simulink model "modelref_s0"  (R2022a)
settings: Solver=FixedStepDiscrete  StartTime=0.0  StopTime=10.0  RelTol=1e-3  EnableMultiTasking=on
model workspace (MAT data in the model file):
  modelws_data = 2
settings Model: DataDictionary=modelref.sldd  Creator=KenYoshioka  LastModifiedBy=KenYoshioka
settings SolverCC: AutoInsertRateTranBlk=on
settings DataIOCC: SaveOutput=off  SaveTime=off
settings OptimizationCC: DefaultParameterBehavior=Inlined  DefaultUnderspecifiedDataType=single  EnhancedBackFolding=on  PassReuseOutputArgsAs=Individual arguments  ZeroExternalMemoryAtStartup=off  ZeroInternalMemoryAtStartup=off  OptimizeBlockOrder=speed  DifferentSizesBufferReuse=on  OptimizationCustomize=off  EfficientTunableParamExpr=on
settings DebuggingCC: ParameterTunabilityLossMsg=error
settings HardwareCC: ProdBitPerPointer=32  ProdBitPerSizeT=32  ProdBitPerPtrDiffT=32  ProdLargestAtomicInteger=Long  ProdLargestAtomicFloat=Double  ProdWordSize=32  ProdHWDeviceType=ARM Compatible->ARM Cortex
settings ModelReferenceCC: ModelReferenceNumInstancesAllowed=Single
settings SFSimCC: MATLABDynamicMemAlloc=off
settings RTWCC: SystemTargetFile=ert.tlc  GenCodeOnly=on  TemplateMakefile=ert_default_tmf  CustomDefine=MBD_REFERENCED_MODEL  Toolchain=GNU Tools for ARM Embedded Processors
settings CodeAppCC: ForceParamTrailComments=on  IgnoreCustomStorageClasses=off  MaxIdLength=255  OperatorAnnotations=on  SimulinkDataObjDesc=on  SFDataObjDesc=on  InsertBlockDesc=on
settings ERTTargetCC: GenerateSampleERTMain=on  InlinedParameterPlacement=NonHierarchical  ERTCustomFileTemplate=example_file_process.tlc

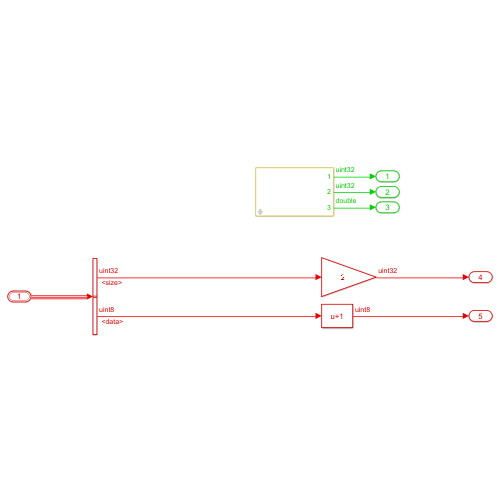
[thumbnail: Simulink's stored preview of the top-level diagram]
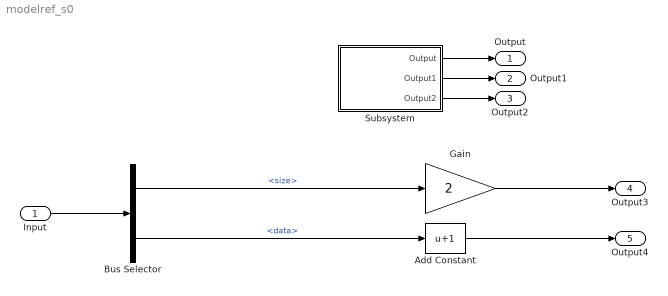
== system modelref_s0 ==
  Input : Inport  OutDataTypeStr=Bus: shared_bus_t
  Add Constant : Bias  Bias=1  SaturateOnIntegerOverflow=off
  Bus Selector : BusSelector  OutputSignals=size,data
  Gain : Gain  Gain=2  OutDataTypeStr=Inherit: Same as input
  Subsystem : Subsystem
      mask init:
      | global Mask_shared_data;
      | if isempty(Mask_shared_data)
      |     disp('(s)Mask_shared_data clear');
      | 
      |     Mask_shared_data = uint32(555);
      | end
      | global Mask_shared_error;
      | 
      | 
      | global Global_signal_index;
      | if isempty(Global_signal_index)
      |     Global_signal_index = uint32(777);
      | end
      | 
      | mws = get_param(bdroot(gcb),'ModelWorkspace');
      | disp('sub');
      | disp(mws.getVariable('modelws_data'));
      | 
      | %Local = evalin('base','mbd.diag');
      | %Local_entry_shared_index = getEntry(Local.ddSec,'shared_index');
      | %Local_param_shared_index = getValue(Local_entry_shared_index);
      | %global Global_shared_index;
      | %Global_shared_index = Local_param_shared_index.Value;
  Output : Outport
  Output1 : Outport  Port=2
  Output2 : Outport  Port=3
  Output3 : Outport  Port=4
  Output4 : Outport  Port=5
  wires:
  Subsystem/1(Output) -> Output/1
  Subsystem/2(Output1) -> Output1/1
  Subsystem/3(Output2) -> Output2/1
  Gain/1 -> Output3/1
  Add Constant/1 -> Output4/1
  Input/1 -> Bus Selector/1
  Bus Selector/1 -> Gain/1  "<size>"
  Bus Selector/2 -> Add Constant/1  "<data>"

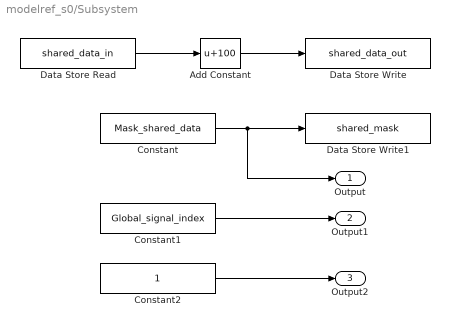
== system modelref_s0/Subsystem ==
  Add Constant : Bias  Bias=100  SaturateOnIntegerOverflow=off
  Constant : Constant  Value=Mask_shared_data  SampleTime=0.01
  Constant1 : Constant  Value=Global_signal_index  SampleTime=0.01
  Constant2 : Constant  SampleTime=0.01
  Data Store Read : DataStoreRead  DataStoreName=shared_data_in  SampleTime=0.001  IndexOptions=Index vector (dialog)  Indices=1  OutputSizes=1
  Data Store Write : DataStoreWrite  DataStoreName=shared_data_out  SampleTime=0.001  IndexOptions=Index vector (dialog)  Indices=1  OutputSizes=1
  Data Store Write1 : DataStoreWrite  DataStoreName=shared_mask  SampleTime=0.01  IndexOptions=Index vector (dialog)  Indices=1  OutputSizes=1
  Output : Outport
  Output1 : Outport  Port=2
  Output2 : Outport  Port=3
  wires:
  Constant/1 -> Output/1, Data Store Write1/1
  Add Constant/1 -> Data Store Write/1
  Data Store Read/1 -> Add Constant/1
  Constant1/1 -> Output1/1
  Constant2/1 -> Output2/1
